simulink model "dlqrest_dist_2x2_2023_2020b"  (R2020b)
settings: Solver=ode23t  StartTime=0.0  StopTime=20  FixedStep=Ts/10  RelTol=1e-8  AbsTol=1e-9
values from neighbouring files (symbols this model uses):
  Bm = 2e-6    (= 2e-06)    [TEST_dist_effect_motor_2023.m]    (also in TestDIST_EFFECT_DCmotor.m = 1.5e-06)
  Festar = Fs-L*[1 0]    [TEST_dist_effect_motor_2023.m]    (also in TestDIST_EFFECT_DCmotor.m)
  Gestar = [Gs L]    [TEST_dist_effect_motor_2023.m]    (also in TestDIST_EFFECT_DCmotor.m)
  Jt = Jm+J1+J2    (= 2.089856e-05)    [TEST_dist_effect_motor_2023.m]    (also in TestDIST_EFFECT_DCmotor.m)
  KK = dlqr(Fs,Gs,Q,R)    [TEST_dist_effect_motor_2023.m]    (also in TestDIST_EFFECT_DCmotor.m)
  Kt = 0.042    [TEST_dist_effect_motor_2023.m]    (also in TestDIST_EFFECT_DCmotor.m)
  Lm = 1.16e-3    (= 0.00116)    [TEST_dist_effect_motor_2023.m]    (also in TestDIST_EFFECT_DCmotor.m)
  Rm = 8.4    [TEST_dist_effect_motor_2023.m]    (also in TestDIST_EFFECT_DCmotor.m)
  Ts = 0.002    [TEST_dist_effect_motor_2023.m]    (also in TestDIST_EFFECT_DCmotor.m)
settings Model: Creator=oboe  LastModifiedBy=Lab-Mec
settings SolverCC: AutoScaleAbsTol=off
settings DataIOCC: ReturnWorkspaceOutputs=off
settings DebuggingCC: ArithmeticOperatorsInVariantConditions=warning
settings SFSimCC: SimUseLocalCustomCode=off  CustomCodeUndefinedFunction=UseInterfaceOnly
settings RTWCC: RTWUseLocalCustomCode=off
settings CodeAppCC: StateflowObjectComments=on

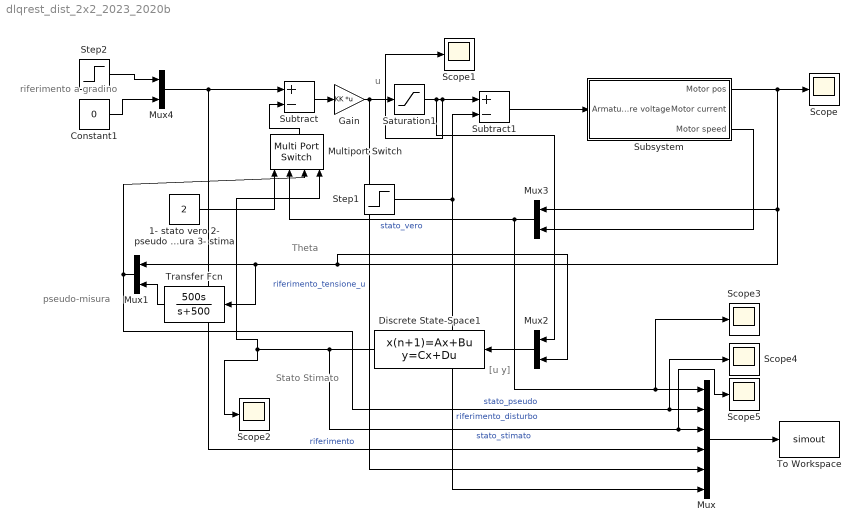
== system dlqrest_dist_2x2_2023_2020b ==
  note: pseudo-misura
  note: [u
      | y]
  note: Stato
      | Stimato
  note: u
  note: Theta
  note: riferimento
      | a gradino
  1- stato vero 2- pseudo misura 3- stima : Constant  Value=2
  Constant1 : Constant  Value=0
  Discrete State-Space1 : DiscreteStateSpace  A=Festar  B=Gestar  C=eye(2)  D=[0 0; 0 0]  InitialCondition=[0 0]'  SampleTime=Ts
  Gain : Gain  Gain=KK  Multiplication=Matrix(K*u)
  Multiport Switch : MultiPortSwitch
  Mux : Mux  Inputs=6
  Mux{1..4} (4 alike) : Mux  Inputs=2
  Saturation1 : Saturate  UpperLimit=6  LowerLimit=-6
  Scope{,1..5} (6 alike) : Scope
  Step1 : Step  Time=3  After=.1  SampleTime=0
  Step2 : Step  SampleTime=0
  Subsystem : Subsystem
  Subtract : Sum  Inputs=+-
  Subtract1 : Sum  Inputs=+-
  To Workspace : ToWorkspace  VariableName=simout  SaveFormat=Structure With Time  SampleTime=-1
  Transfer Fcn : TransferFcn  Numerator=[500 0]  Denominator=[1 500]
  wires:
  Subtract/1 -> Gain/1
  Subsystem/1(Motor pos) -> Mux2/2, Transfer Fcn/1, Mux1/1, Mux3/1, Scope/1
  Transfer Fcn/1 -> Mux1/2
  Mux2/1 -> Discrete State-Space1/1
  Mux1/1 -> Multiport Switch/3, Scope4/1, Mux/2  "stato_pseudo"
  1- stato vero 2- pseudo misura 3- stima/1 -> Multiport Switch/1
  Multiport Switch/1 -> Subtract/2
  Saturation1/1 -> Scope1/1, Subtract1/1, Mux2/1
  Step1/1 -> Mux/6, Subtract1/2  "riferimento_disturbo"
  Gain/1 -> Mux/5, Saturation1/1  "riferimento_tensione_u"
  Discrete State-Space1/1 -> Scope5/1, Mux/3, Multiport Switch/4, Scope2/1  "stato_stimato"
  Constant1/1 -> Mux4/2
  Step2/1 -> Mux4/1
  Mux4/1 -> Mux/4, Subtract/1  "riferimento"
  Subtract1/1 -> Subsystem/1(Armature voltage)
  Mux3/1 -> Multiport Switch/2, Scope3/1, Mux/1  "stato_vero"
  Subsystem/3(Motor speed) -> Mux3/2
  Mux/1 -> To Workspace/1

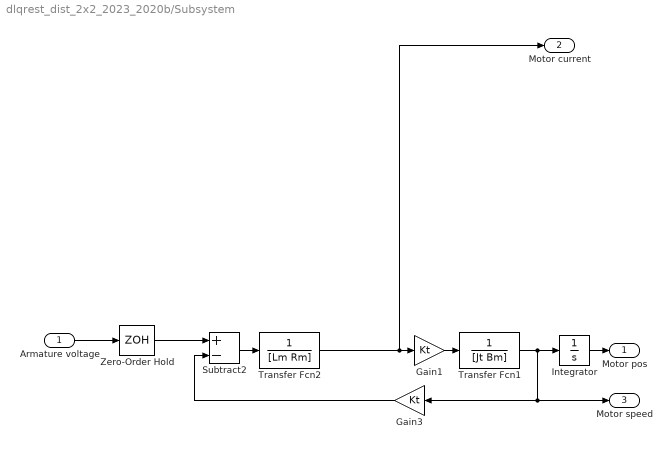
== system dlqrest_dist_2x2_2023_2020b/Subsystem ==
  Armature voltage : Inport
  Gain1 : Gain  Gain=Kt
  Gain3 : Gain  Gain=Kt
  Integrator : Integrator
  Subtract2 : Sum  Inputs=+-
  Transfer Fcn1 : TransferFcn  Denominator=[Jt Bm]
  Transfer Fcn2 : TransferFcn  Denominator=[Lm Rm]
  Zero-Order Hold : ZeroOrderHold  SampleTime=.002
  Motor pos : Outport
  Motor current : Outport  Port=2
  Motor speed : Outport  Port=3
  wires:
  Integrator/1 -> Motor pos/1
  Zero-Order Hold/1 -> Subtract2/1
  Gain1/1 -> Transfer Fcn1/1
  Transfer Fcn2/1 -> Motor current/1, Gain1/1
  Gain3/1 -> Subtract2/2
  Subtract2/1 -> Transfer Fcn2/1
  Armature voltage/1 -> Zero-Order Hold/1
  Transfer Fcn1/1 -> Motor speed/1, Gain3/1, Integrator/1
